simulink model "sine_gen_triphase_v3"  (R2025a)
settings: Solver=VariableStepAuto  StartTime=0.0  StopTime=2e-4  RelTol=1e-3
model workspace (MAT data in the model file):
  NoaFutureIOMap{1}.PortName = 'amp'
  NoaFutureIOMap{1}.PortType = 'Inport'
  NoaFutureIOMap{1}.DataType = 'sfix32_En21'
  NoaFutureIOMap{1}.IOInterface = 'AXI4-Lite'
  NoaFutureIOMap{1}.IOInterfaceMapping = 'x"100"'
  NoaFutureIOMap{2}.PortName = 'freq'
  NoaFutureIOMap{2}.PortType = 'Inport'
  NoaFutureIOMap{2}.DataType = 'uint32'
  NoaFutureIOMap{2}.IOInterface = 'AXI4-Lite'
  NoaFutureIOMap{2}.IOInterfaceMapping = 'x"104"'
  NoaFutureIOMap{3}.PortName = 'sine_phase1'
  NoaFutureIOMap{3}.PortType = 'Outport'
  NoaFutureIOMap{3}.DataType = 'sfix32_En21'
  NoaFutureIOMap{3}.IOInterface = 'DAQ Channel 0 [0:31]'
  NoaFutureIOMap{3}.IOInterfaceMapping = '[0:31]'
  NoaFutureIOMap{4}.PortName = 'sine_analog1'
  NoaFutureIOMap{4}.PortType = 'Outport'
  NoaFutureIOMap{4}.DataType = 'sfix32_En23'
  NoaFutureIOMap{4}.IOInterface = 'Analog Output 0 [0:31]'
  NoaFutureIOMap{4}.IOInterfaceMapping = '[0:31]'
  NoaFutureIOMap{4}.NoaBlockParameters.SignalMin = '-300'
  NoaFutureIOMap{4}.NoaBlockParameters.SignalMax = '300'
  NoaFutureIOMap{4}.NoaBlockParameters.VoltageMin = '-3'
  NoaFutureIOMap{4}.NoaBlockParameters.VoltageMax = '3'
  NoaFutureIOMap{4}.NoaBlockParameters.LUT_Signals = '[-300 -240 -180 -120  -60    0   60  120  180  240  300]'
  NoaFutureIOMap{4}.NoaBlockParameters.LUT_Values = '[-3        -2.4        -1.8        -1.2        -0.6           0         0.6         1.2         1.8         2.4           3]'
  NoaFutureIOMap{5}.PortName = 'sine_phase2'
  NoaFutureIOMap{5}.PortType = 'Outport'
  NoaFutureIOMap{5}.DataType = 'sfix32_En21'
  NoaFutureIOMap{5}.IOInterface = 'DAQ Channel 1 [0:31]'
  NoaFutureIOMap{5}.IOInterfaceMapping = '[0:31]'
  NoaFutureIOMap{6}.PortName = 'sine_analog2'
  NoaFutureIOMap{6}.PortType = 'Outport'
  NoaFutureIOMap{6}.DataType = 'sfix32_En23'
  NoaFutureIOMap{6}.IOInterface = 'Analog Output 1 [0:31]'
  NoaFutureIOMap{6}.IOInterfaceMapping = '[0:31]'
  NoaFutureIOMap{6}.NoaBlockParameters.SignalMin = '-300'
  NoaFutureIOMap{6}.NoaBlockParameters.SignalMax = '300'
  NoaFutureIOMap{6}.NoaBlockParameters.VoltageMin = '-3'
  NoaFutureIOMap{6}.NoaBlockParameters.VoltageMax = '3'
  NoaFutureIOMap{6}.NoaBlockParameters.LUT_Signals = '[-300 -240 -180 -120  -60    0   60  120  180  240  300]'
  NoaFutureIOMap{6}.NoaBlockParameters.LUT_Values = '[-3        -2.4        -1.8        -1.2        -0.6           0         0.6         1.2         1.8         2.4           3]'
  NoaFutureIOMap{7}.PortName = 'sine_phase3'
  NoaFutureIOMap{7}.PortType = 'Outport'
  NoaFutureIOMap{7}.DataType = 'sfix32_En21'
  NoaFutureIOMap{7}.IOInterface = 'DAQ Channel 2 [0:31]'
  NoaFutureIOMap{7}.IOInterfaceMapping = '[0:31]'
  NoaFutureIOMap{8}.PortName = 'sine_analog3'
  NoaFutureIOMap{8}.PortType = 'Outport'
  NoaFutureIOMap{8}.DataType = 'sfix32_En23'
  NoaFutureIOMap{8}.IOInterface = 'Analog Output 2 [0:31]'
  NoaFutureIOMap{8}.IOInterfaceMapping = '[0:31]'
  NoaFutureIOMap{8}.NoaBlockParameters.SignalMin = '-300'
  NoaFutureIOMap{8}.NoaBlockParameters.SignalMax = '300'
  NoaFutureIOMap{8}.NoaBlockParameters.VoltageMin = '-3'
  NoaFutureIOMap{8}.NoaBlockParameters.VoltageMax = '3'
  NoaFutureIOMap{8}.NoaBlockParameters.LUT_Signals = '[-300 -240 -180 -120  -60    0   60  120  180  240  300]'
  NoaFutureIOMap{8}.NoaBlockParameters.LUT_Values = '[-3        -2.4        -1.8        -1.2        -0.6           0         0.6         1.2         1.8         2.4           3]'
undefined symbols (not defined in the file): period
libraries: hdlsllib x12, library_AnalogOut x3
settings Model: Creator=tarko  LastModifiedBy=ambre
settings OptimizationCC: BlockReduction=off  ConditionallyExecuteInputs=off  DefaultParameterBehavior=Inlined
settings DebuggingCC: AlgebraicLoopMsg=error
settings HardwareCC: ProdBitPerPointer=32.0  ProdBitPerSizeT=32.0  ProdBitPerPtrDiffT=32.0  ProdLargestAtomicFloat=None  ProdIntDivRoundTo=Undefined  ProdEndianess=Unspecified  ProdWordSize=32.0  ProdHWDeviceType=ASIC/FPGA->ASIC/FPGA  TargetBitPerPointer=64.0  TargetBitPerSizeT=64.0  TargetBitPerPtrDiffT=64.0  TargetLongLongMode=on  TargetIntDivRoundTo=Zero  TargetEndianess=LittleEndian  TargetWordSize=64.0  TargetHWDeviceType=Custom Processor->MATLAB Host Computer  ProdEqTarget=off

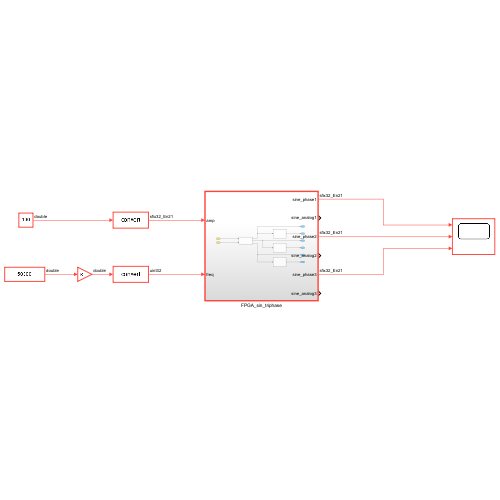
[thumbnail: Simulink's stored preview of the top-level diagram]
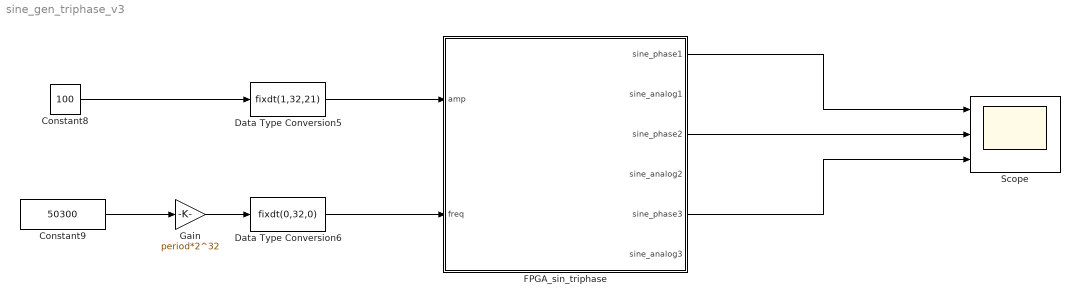
== system sine_gen_triphase_v3 ==
  Constant8 : Constant  Value=100  SampleTime=period
  Constant9 : Constant  Value=50300  SampleTime=period
  Data Type Conversion5 : DataTypeConversion  OutDataTypeStr=fixdt(1,32,21)  SaturateOnIntegerOverflow=off  RndMeth=Floor
  Data Type Conversion6 : DataTypeConversion  OutDataTypeStr=fixdt(0,32,0)  SaturateOnIntegerOverflow=off  RndMeth=Floor
  FPGA_sin_triphase : Subsystem  TreatAsAtomicUnit=on
  Gain : Gain  Gain=period*2^32
  Scope : Scope  NumInputPorts=3
      settings: ActiveDisplayYMinimum=-125  ActiveDisplayYMaximum=125
  wires:
  Constant8/1 -> Data Type Conversion5/1
  Constant9/1 -> Gain/1
  Gain/1 -> Data Type Conversion6/1
  Data Type Conversion5/1 -> FPGA_sin_triphase/1(amp)
  Data Type Conversion6/1 -> FPGA_sin_triphase/2(freq)
  FPGA_sin_triphase/1(sine_phase1) -> Scope/1
  FPGA_sin_triphase/3(sine_phase2) -> Scope/2
  FPGA_sin_triphase/5(sine_phase3) -> Scope/3

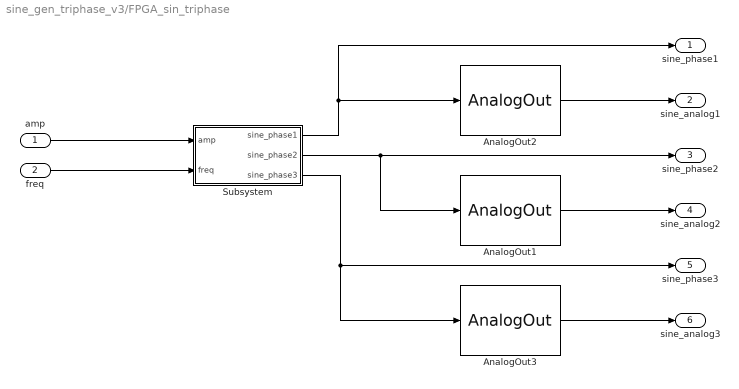
== system sine_gen_triphase_v3/FPGA_sin_triphase ==
  amp : Inport
  freq : Inport  Port=2
  AnalogOut1 : library_AnalogOut/AnalogOut  SignalMin=-300  SignalMax=300  VoltageMin=-3  VoltageMax=3
  AnalogOut2 : library_AnalogOut/AnalogOut  SignalMin=-300  SignalMax=300  VoltageMin=-3  VoltageMax=3
  AnalogOut3 : library_AnalogOut/AnalogOut  SignalMin=-300  SignalMax=300  VoltageMin=-3  VoltageMax=3
  Subsystem : Subsystem
  sine_phase1 : Outport
  sine_analog1 : Outport  Port=2
  sine_phase2 : Outport  Port=3
  sine_analog2 : Outport  Port=4
  sine_phase3 : Outport  Port=5
  sine_analog3 : Outport  Port=6
  wires:
  Subsystem/1(sine_phase1) -> AnalogOut2/1, sine_phase1/1
  amp/1 -> Subsystem/1(amp)
  freq/1 -> Subsystem/2(freq)
  AnalogOut2/1 -> sine_analog1/1
  AnalogOut1/1 -> sine_analog2/1
  AnalogOut3/1 -> sine_analog3/1
  Subsystem/2(sine_phase2) -> sine_phase2/1, AnalogOut1/1
  Subsystem/3(sine_phase3) -> sine_phase3/1, AnalogOut3/1

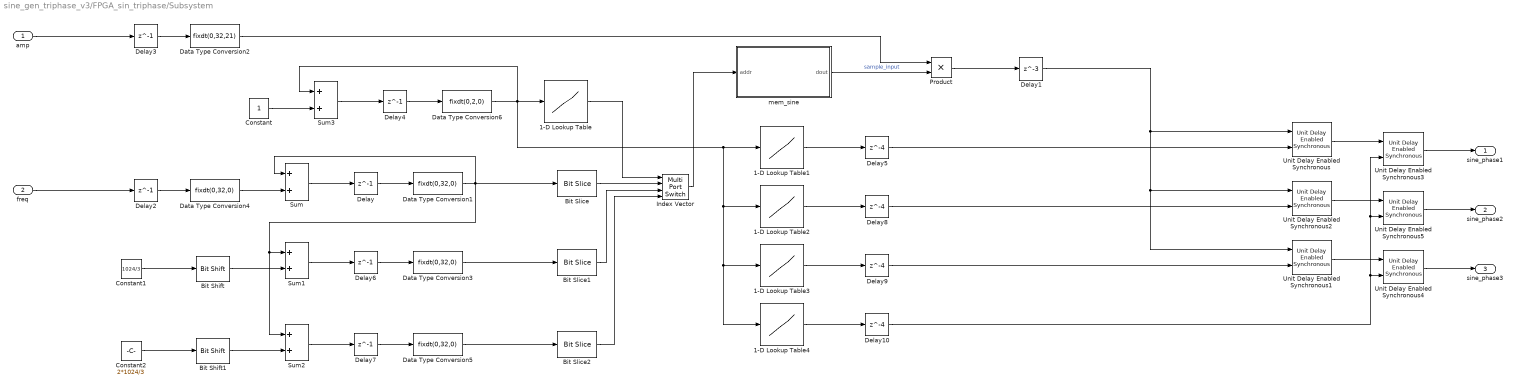
== system sine_gen_triphase_v3/FPGA_sin_triphase/Subsystem ==
  amp : Inport
  freq : Inport  Port=2
  1-D Lookup Table : Lookup_n-D  NumberOfTableDimensions=1  LookupTableObject=''  BreakpointsForDimension1=[0:3]  BreakpointsForDimension1FirstPoint=10  BreakpointsForDimension2FirstPoint=10  BreakpointsForDimension1Spacing=12  BreakpointsForDimension2Spacing=12  IndexSearchMethod=Evenly spaced points  Table=[0 1 2 0]  InterpMethod=Flat  DiagnosticForOutOfRangeInput=Error  InternalRulePriority=Speed  OutDataTypeStr=fixdt(0,2,0)  RndMeth=Simplest
  1-D Lookup Table1 : Lookup_n-D  NumberOfTableDimensions=1  LookupTableObject=''  BreakpointsForDimension1=[0:3]  BreakpointsForDimension1FirstPoint=10  BreakpointsForDimension2FirstPoint=10  BreakpointsForDimension1Spacing=12  BreakpointsForDimension2Spacing=12  IndexSearchMethod=Evenly spaced points  Table=[1 0 0 0]  InterpMethod=Flat  DiagnosticForOutOfRangeInput=Error  InternalRulePriority=Speed  OutDataTypeStr=fixdt(0,1,0)  RndMeth=Simplest
  1-D Lookup Table2 : Lookup_n-D  NumberOfTableDimensions=1  LookupTableObject=''  BreakpointsForDimension1=[0:3]  BreakpointsForDimension1FirstPoint=10  BreakpointsForDimension2FirstPoint=10  BreakpointsForDimension1Spacing=12  BreakpointsForDimension2Spacing=12  IndexSearchMethod=Evenly spaced points  Table=[0 1 0 0]  InterpMethod=Flat  DiagnosticForOutOfRangeInput=Error  InternalRulePriority=Speed  OutDataTypeStr=fixdt(0,1,0)  RndMeth=Simplest
  1-D Lookup Table3 : Lookup_n-D  NumberOfTableDimensions=1  LookupTableObject=''  BreakpointsForDimension1=[0:3]  BreakpointsForDimension1FirstPoint=10  BreakpointsForDimension2FirstPoint=10  BreakpointsForDimension1Spacing=12  BreakpointsForDimension2Spacing=12  IndexSearchMethod=Evenly spaced points  Table=[0 0 1 0]  InterpMethod=Flat  DiagnosticForOutOfRangeInput=Error  InternalRulePriority=Speed  OutDataTypeStr=fixdt(0,1,0)  RndMeth=Simplest
  1-D Lookup Table4 : Lookup_n-D  NumberOfTableDimensions=1  LookupTableObject=''  BreakpointsForDimension1=[0:3]  BreakpointsForDimension1FirstPoint=10  BreakpointsForDimension2FirstPoint=10  BreakpointsForDimension1Spacing=12  BreakpointsForDimension2Spacing=12  IndexSearchMethod=Evenly spaced points  Table=[0 0 0 1]  InterpMethod=Flat  DiagnosticForOutOfRangeInput=Error  InternalRulePriority=Speed  OutDataTypeStr=fixdt(0,1,0)  RndMeth=Simplest
  Bit Shift : hdlsllib/Logic and Bit Operations/Bit Shift  mode=Shift Left Logical  N=22
  Bit Shift1 : hdlsllib/Logic and Bit Operations/Bit Shift  mode=Shift Left Logical  N=22
  Bit Slice : hdlsllib/Logic and Bit Operations/Bit Slice  lidx=31  ridx=22
  Bit Slice1 : hdlsllib/Logic and Bit Operations/Bit Slice  lidx=31  ridx=22
  Bit Slice2 : hdlsllib/Logic and Bit Operations/Bit Slice  lidx=31  ridx=22
  Constant : Constant  OutDataTypeStr=fixdt(0,2,0)
  Constant1 : Constant  Value=1024/3  OutDataTypeStr=uint32  SampleTime=period
  Constant2 : Constant  Value=2*1024/3  OutDataTypeStr=uint32  SampleTime=period
  Data Type Conversion{1,3..5} (4 alike) : DataTypeConversion  OutDataTypeStr=fixdt(0,32,0)  SaturateOnIntegerOverflow=off  RndMeth=Floor
  Data Type Conversion2 : DataTypeConversion  OutDataTypeStr=fixdt(0,32,21)  SaturateOnIntegerOverflow=off  RndMeth=Floor
  Data Type Conversion6 : DataTypeConversion  OutDataTypeStr=fixdt(0,2,0)  SaturateOnIntegerOverflow=off  RndMeth=Floor
  Delay{,4,6..7} (4 alike) : Delay  DelayLength=1  InitialCondition=0
  Delay1 : Delay  DelayLength=3  InitialCondition=0
  Delay{5,8..10} (4 alike) : Delay  DelayLength=4  InitialCondition=1
  Delay2 : Delay  DelayLength=1  InitialCondition=(50300*period)*2^32
  Delay3 : Delay  DelayLength=1  InitialCondition=100
  Index Vector : MultiPortSwitch  DataPortOrder=Zero-based contiguous  zeroidx=on  SaturateOnIntegerOverflow=off  InputSameDT=off
  Product : Product  OutDataTypeStr=fixdt(1,32,21)
  Sum : Sum  OutDataTypeStr=uint32
  Sum1 : Sum  OutDataTypeStr=uint32
  Sum2 : Sum  OutDataTypeStr=uint32
  Sum3 : Sum  OutDataTypeStr=fixdt(0,2,0)
  Unit Delay Enabled Synchronous{,1..5} (6 alike) : hdlsllib/Discrete/Unit Delay Enabled Synchronous  InitialCondition=0.0  SampleTime=-1
  mem_sine : Subsystem  mask{data=sin(2*pi*(0:1023)/1024), bw=32}
      mask prompts: data "Initial Data"; bw "Bitwidth"
  sine_phase1 : Outport
  sine_phase2 : Outport  Port=2
  sine_phase3 : Outport  Port=3
  wires:
  freq/1 -> Delay2/1
  Data Type Conversion2/1 -> Product/1
  Delay/1 -> Data Type Conversion1/1
  Data Type Conversion1/1 -> Sum2/1, Sum1/1, Sum/1, Bit Slice/1
  Data Type Conversion4/1 -> Sum/2
  Delay3/1 -> Data Type Conversion2/1
  mem_sine/1(dout) -> Product/2  "sample_input"
  Sum/1 -> Delay/1
  Delay2/1 -> Data Type Conversion4/1
  Product/1 -> Delay1/1
  amp/1 -> Delay3/1
  Data Type Conversion3/1 -> Bit Slice1/1
  Delay6/1 -> Data Type Conversion3/1
  Sum1/1 -> Delay6/1
  Data Type Conversion5/1 -> Bit Slice2/1
  Delay7/1 -> Data Type Conversion5/1
  Sum2/1 -> Delay7/1
  Bit Slice/1 -> Index Vector/2
  Bit Slice1/1 -> Index Vector/3
  Bit Slice2/1 -> Index Vector/4
  Index Vector/1 -> mem_sine/1(addr)
  Delay1/1 -> Unit Delay Enabled Synchronous1/1, Unit Delay Enabled Synchronous2/1, Unit Delay Enabled Synchronous/1
  Constant/1 -> Sum3/2
  Data Type Conversion6/1 -> 1-D Lookup Table2/1, 1-D Lookup Table3/1, 1-D Lookup Table4/1, 1-D Lookup Table1/1, 1-D Lookup Table/1, Sum3/1
  Delay4/1 -> Data Type Conversion6/1
  Sum3/1 -> Delay4/1
  1-D Lookup Table/1 -> Index Vector/1
  1-D Lookup Table1/1 -> Delay5/1
  1-D Lookup Table2/1 -> Delay8/1
  1-D Lookup Table3/1 -> Delay9/1
  Delay5/1 -> Unit Delay Enabled Synchronous/2
  Delay8/1 -> Unit Delay Enabled Synchronous2/2
  Delay9/1 -> Unit Delay Enabled Synchronous1/2
  Unit Delay Enabled Synchronous/1 -> Unit Delay Enabled Synchronous3/1
  Unit Delay Enabled Synchronous2/1 -> Unit Delay Enabled Synchronous5/1
  Unit Delay Enabled Synchronous1/1 -> Unit Delay Enabled Synchronous4/1
  Unit Delay Enabled Synchronous3/1 -> sine_phase1/1
  Unit Delay Enabled Synchronous5/1 -> sine_phase2/1
  Unit Delay Enabled Synchronous4/1 -> sine_phase3/1
  1-D Lookup Table4/1 -> Delay10/1
  Delay10/1 -> Unit Delay Enabled Synchronous3/2, Unit Delay Enabled Synchronous5/2, Unit Delay Enabled Synchronous4/2
  Constant1/1 -> Bit Shift/1
  Bit Shift/1 -> Sum1/2
  Constant2/1 -> Bit Shift1/1
  Bit Shift1/1 -> Sum2/2

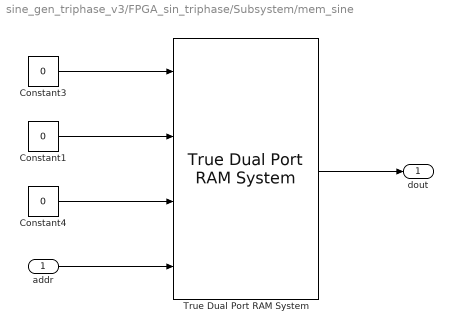
== system sine_gen_triphase_v3/FPGA_sin_triphase/Subsystem/mem_sine ==
  addr : Inport
  Constant1 : Constant  Value=0  OutDataTypeStr=fixdt(0,10,0)  SampleTime=period
  Constant3 : Constant  Value=0  OutDataTypeStr=fixdt(1,bw,21)  SampleTime=period
  Constant4 : Constant  Value=0  OutDataTypeStr=boolean  SampleTime=period
  True Dual Port RAM System : hdlsllib/HDL RAMs/True Dual Port RAM System  RAMType=Simple dual port  AsyncRead=off  WriteOutputValue=Old data  RAMInitialValue=data  allowBusInputs=off  WritesHaveOutput=on  NumReads=0  NumWrites=1  SimulateUsing=Code generation  ModelRAMDelay=on  VectorAccess=Parallel
  dout : Outport
  wires:
  True Dual Port RAM System/1 -> dout/1
  Constant1/1 -> True Dual Port RAM System/2
  Constant3/1 -> True Dual Port RAM System/1
  Constant4/1 -> True Dual Port RAM System/3
  addr/1 -> True Dual Port RAM System/4
